simulink model "impedanceExperiments"  (R2019a)
settings: Solver=ode4  StartTime=0.0  StopTime=30  FixedStep=0.01  RelTol=1e-3
libraries: dspswit3 x2
settings Model: Creator=JanAriel  LastModifiedBy=JanAriel
settings SolverCC: AlgebraicLoopSolver=LineSearch

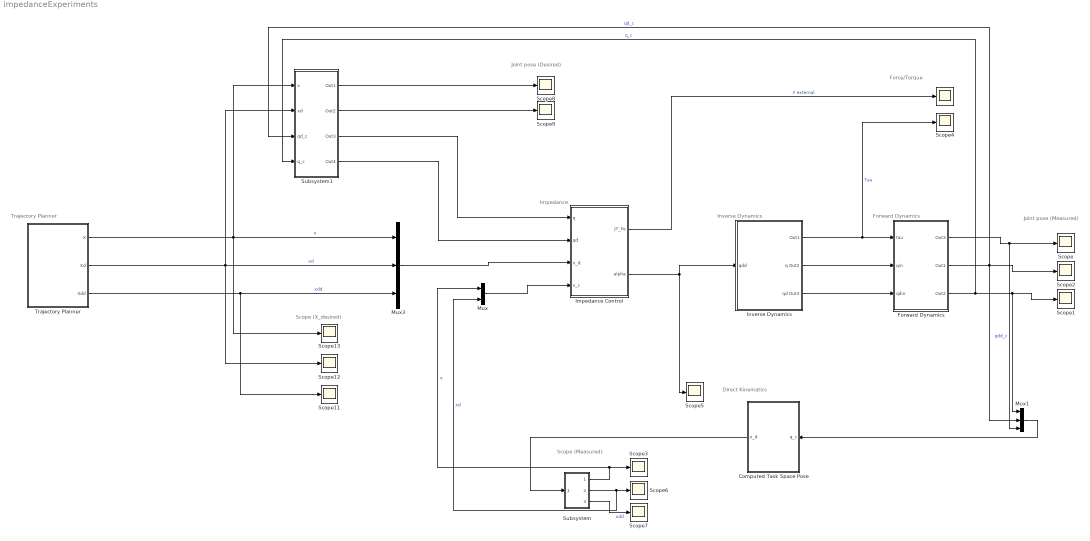
== system impedanceExperiments ==
  note: Joint pose (Desired)
  note: Force/Torque
  note: Joint pose (Measured)
  note: Scope (X_desired)
  note: Scope (Measured)
  note: Trajectory Planner
  note: Forward Dynamics
  note: Inverse Dynamics
  note: Direct Kinematics
  note: Impedance
  " " : Scope
  Computed Task Space Pose : Subsystem
  Forward Dynamics : Subsystem
  Impedance Control : Subsystem
  Inverse Dynamics : Subsystem
  Mux : Mux  Inputs=2
  Mux1 : Mux  Inputs=3
  Mux3 : Mux  Inputs=3
  Scope{,1..9,11..13} (13 alike) : Scope
  Subsystem : Subsystem
  Subsystem1 : Subsystem
  Trajectory Planner : Subsystem
  wires:
  Inverse Dynamics/1(Out1) -> Forward Dynamics/1(tau), Scope4/1  "Tau"
  Inverse Dynamics/2(q Out2) -> Forward Dynamics/2(qin)
  Forward Dynamics/3(Out2) -> Subsystem1/4(q_c), Mux1/1, Scope1/1  "q_c"
  Forward Dynamics/1(Out3) -> Scope/1, Mux1/3  "qdd_c"
  Forward Dynamics/2(Out1) -> Subsystem1/3(qd_c), Mux1/2, Scope2/1  "qd_c"
  Impedance Control/1(JT_Fe) -> " "/1  "F external"
  Trajectory Planner/1(X) -> Subsystem1/1(x), Mux3/1, Scope13/1  "x"
  Trajectory Planner/2(Xd) -> Scope12/1, Mux3/2, Subsystem1/2(xd)  "xd"
  Trajectory Planner/3(Xdd) -> Scope11/1, Mux3/3  "xdd"
  Mux3/1 -> Impedance Control/3(x_d)
  Inverse Dynamics/3(qd Out3) -> Forward Dynamics/3(qdin)
  Computed Task Space Pose/1(x_d) -> Subsystem/1(In1)
  Mux1/1 -> Computed Task Space Pose/1(q_c)
  Impedance Control/2(alpha) -> Scope5/1, Inverse Dynamics/1(qdd)
  Subsystem/1(Out1) -> Scope3/1, Mux/1  "x"
  Subsystem/2(Out2) -> Mux/2, Scope6/1  "xd"
  Subsystem/3(Out3) -> Scope7/1  "xdd"
  Mux/1 -> Impedance Control/4(x_c)
  Subsystem1/1(Out1) -> Scope8/1
  Subsystem1/2(Out2) -> Scope9/1
  Subsystem1/3(Out3) -> Impedance Control/1(q)
  Subsystem1/4(Out4) -> Impedance Control/2(qd)

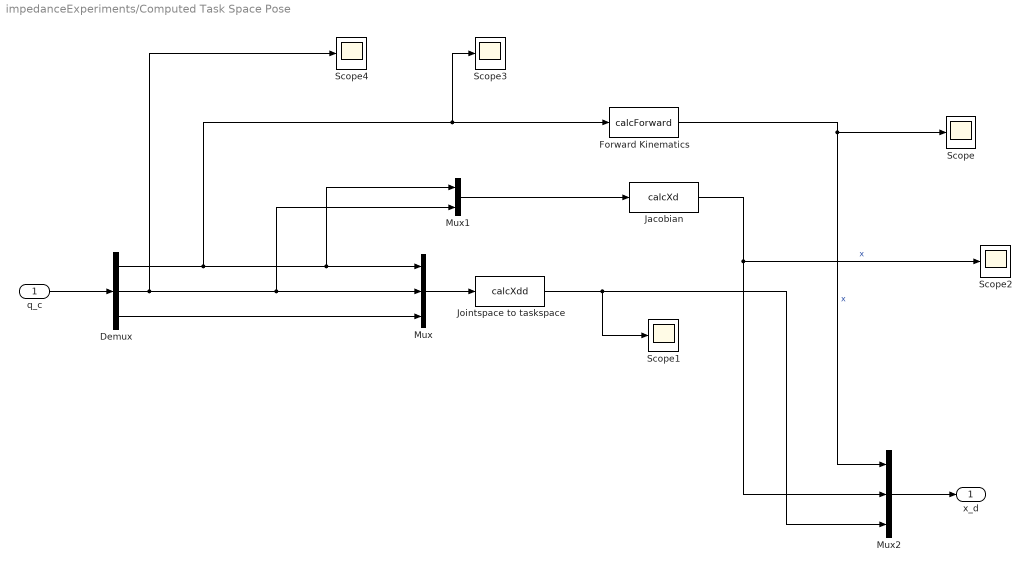
== system impedanceExperiments/Computed Task Space Pose ==
  q_c : Inport
  Demux : Demux  Outputs=3
  Forward Kinematics : MATLABFcn  MATLABFcn=calcForward  Output1D=off
  Jacobian : MATLABFcn  MATLABFcn=calcXd  Output1D=off
  Jointspace to taskspace : MATLABFcn  MATLABFcn=calcXdd  Output1D=off
  Mux : Mux  Inputs=3
  Mux1 : Mux  Inputs=2
  Mux2 : Mux  Inputs=3
  Scope{,1..4} (5 alike) : Scope
  x_d : Outport
  wires:
  q_c/1 -> Demux/1
  Mux/1 -> Jointspace to taskspace/1
  Demux/2 -> Scope4/1, Mux/2, Mux1/2
  Forward Kinematics/1 -> Mux2/1, Scope/1  "x"
  Demux/1 -> Scope3/1, Forward Kinematics/1, Mux/1, Mux1/1
  Mux1/1 -> Jacobian/1
  Demux/3 -> Mux/3
  Jointspace to taskspace/1 -> Scope1/1, Mux2/3
  Mux2/1 -> x_d/1
  Jacobian/1 -> Scope2/1, Mux2/2  "x"

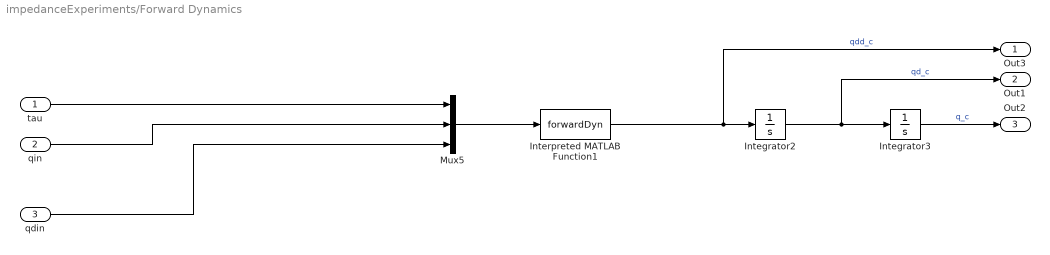
== system impedanceExperiments/Forward Dynamics ==
  tau : Inport
  qin : Inport  Port=2
  qdin : Inport  Port=3
  Integrator2 : Integrator
  Integrator3 : Integrator
  Interpreted MATLAB Function1 : MATLABFcn  MATLABFcn=forwardDyn  Output1D=off
  Mux5 : Mux  Inputs=3
  Out3 : Outport
  Out1 : Outport  Port=2
  Out2 : Outport  Port=3
  wires:
  Integrator2/1 -> Integrator3/1, Out1/1  "qd_c"
  Integrator3/1 -> Out2/1  "q_c"
  Interpreted MATLAB Function1/1 -> Out3/1, Integrator2/1  "qdd_c"
  tau/1 -> Mux5/1
  qin/1 -> Mux5/2
  qdin/1 -> Mux5/3
  Mux5/1 -> Interpreted MATLAB Function1/1

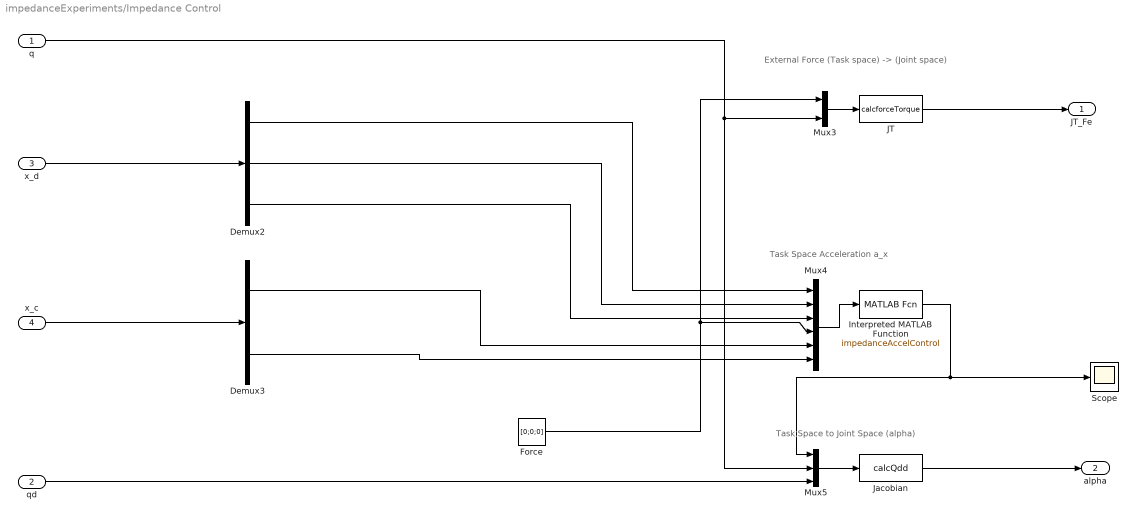
== system impedanceExperiments/Impedance Control ==
  note: Task Space to Joint Space (alpha)
  note: Task Space Acceleration a_x
  note: External Force (Task space) -> (Joint space)
  q : Inport
  qd : Inport  Port=2
  x_d : Inport  Port=3
  x_c : Inport  Port=4
  Demux2 : Demux  Outputs=3
  Demux3 : Demux  Outputs=2
  Force : Constant  Value=[0;0;0]
  Interpreted MATLAB Function : MATLABFcn  MATLABFcn=impedanceAccelControl  Output1D=off
  JT : MATLABFcn  MATLABFcn=calcforceTorque  Output1D=off
  Jacobian : MATLABFcn  MATLABFcn=calcQdd  Output1D=off
  Mux3 : Mux  Inputs=2
  Mux4 : Mux  Inputs=6
  Mux5 : Mux  Inputs=3
  Scope : Scope
  JT_Fe : Outport
  alpha : Outport  Port=2
  wires:
  Demux2/2 -> Mux4/2
  Mux3/1 -> JT/1
  JT/1 -> JT_Fe/1
  Demux2/1 -> Mux4/1
  Demux2/3 -> Mux4/3
  Mux4/1 -> Interpreted MATLAB Function/1
  q/1 -> Mux3/2, Mux5/2
  Mux5/1 -> Jacobian/1
  Interpreted MATLAB Function/1 -> Mux5/1, Scope/1
  Jacobian/1 -> alpha/1
  qd/1 -> Mux5/3
  x_d/1 -> Demux2/1
  Demux3/1 -> Mux4/5
  Demux3/2 -> Mux4/6
  x_c/1 -> Demux3/1
  Force/1 -> Mux3/1, Mux4/4

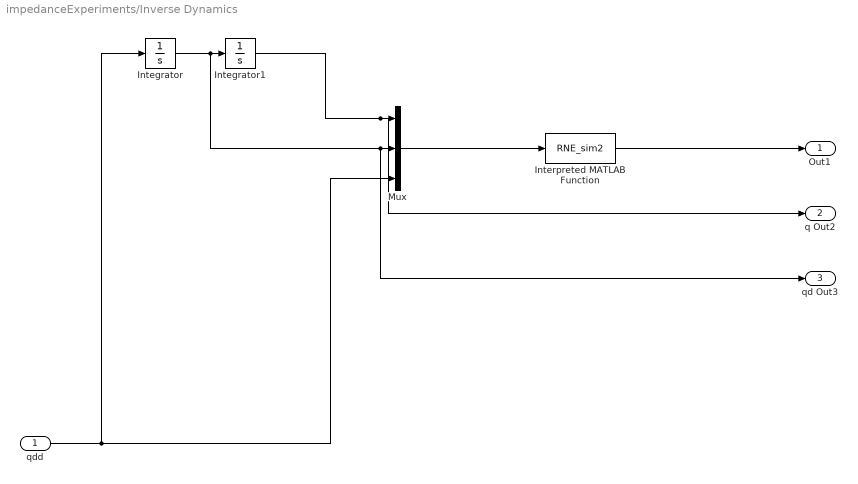
== system impedanceExperiments/Inverse Dynamics ==
  qdd : Inport
  Integrator : Integrator
  Integrator1 : Integrator
  Interpreted MATLAB Function : MATLABFcn  MATLABFcn=RNE_sim2  Output1D=off
  Mux : Mux  Inputs=3
  Out1 : Outport
  q Out2 : Outport  Port=2
  qd Out3 : Outport  Port=3
  wires:
  Mux/1 -> Interpreted MATLAB Function/1
  Interpreted MATLAB Function/1 -> Out1/1
  qdd/1 -> Integrator/1, Mux/3
  Integrator/1 -> qd Out3/1, Mux/2, Integrator1/1
  Integrator1/1 -> q Out2/1, Mux/1

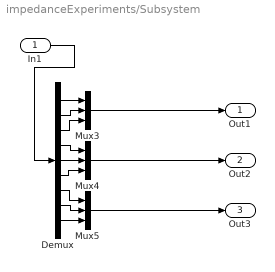
== system impedanceExperiments/Subsystem ==
  In1 : Inport
  Demux : Demux  Outputs=9
  Mux3 : Mux  Inputs=3
  Mux4 : Mux  Inputs=3
  Mux5 : Mux  Inputs=3
  Out1 : Outport
  Out2 : Outport  Port=2
  Out3 : Outport  Port=3
  wires:
  Demux/8 -> Mux5/2
  Demux/7 -> Mux5/1
  Demux/1 -> Mux3/1
  Demux/3 -> Mux3/3
  Demux/9 -> Mux5/3
  Demux/6 -> Mux4/3
  Demux/5 -> Mux4/2
  Demux/4 -> Mux4/1
  Demux/2 -> Mux3/2
  Mux5/1 -> Out3/1
  In1/1 -> Demux/1
  Mux4/1 -> Out2/1
  Mux3/1 -> Out1/1

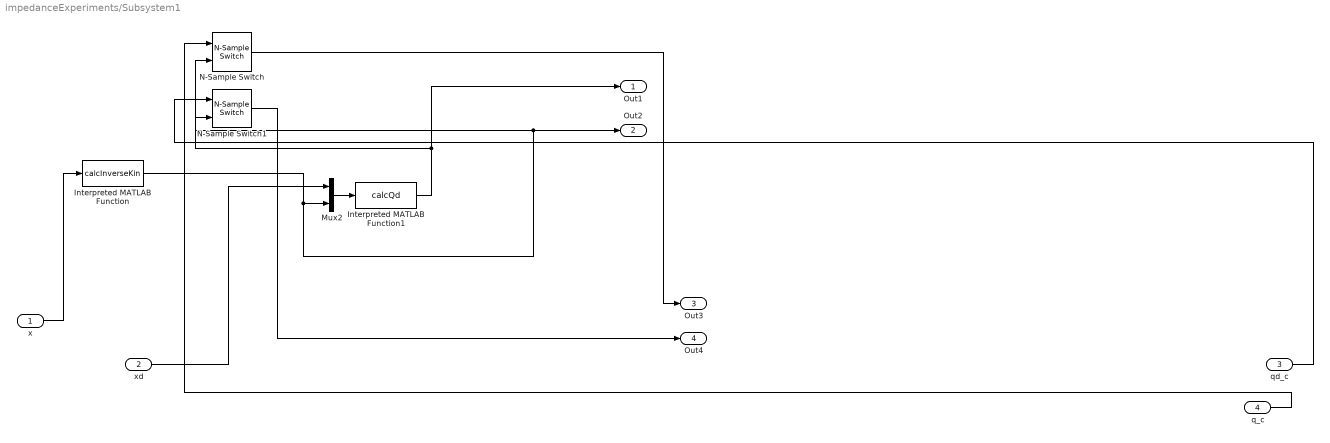
== system impedanceExperiments/Subsystem1 ==
  x : Inport
  xd : Inport  Port=2
  qd_c : Inport  Port=3
  q_c : Inport  Port=4
  Interpreted MATLAB Function : MATLABFcn  MATLABFcn=calcInverseKin  Output1D=off
  Interpreted MATLAB Function1 : MATLABFcn  MATLABFcn=calcQd  Output1D=off
  Mux2 : Mux  Inputs=2
  N-Sample Switch : dspswit3/N-Sample Switch  N=1  reset=off  TriggerType=Rising edge  Ts=0.03
      settings: SourceProductName=DSP System Toolbox  SourceProductBaseCode=DS
  N-Sample Switch1 : dspswit3/N-Sample Switch  N=1  reset=off  TriggerType=Rising edge  Ts=0.03
      settings: SourceProductName=DSP System Toolbox  SourceProductBaseCode=DS
  Out1 : Outport
  Out2 : Outport  Port=2
  Out3 : Outport  Port=3
  Out4 : Outport  Port=4
  wires:
  xd/1 -> Mux2/1
  Interpreted MATLAB Function1/1 -> Out1/1, N-Sample Switch1/2
  N-Sample Switch1/1 -> Out4/1
  Interpreted MATLAB Function/1 -> Out2/1, N-Sample Switch/2, Mux2/2
  Mux2/1 -> Interpreted MATLAB Function1/1
  qd_c/1 -> N-Sample Switch1/1
  N-Sample Switch/1 -> Out3/1
  x/1 -> Interpreted MATLAB Function/1
  q_c/1 -> N-Sample Switch/1

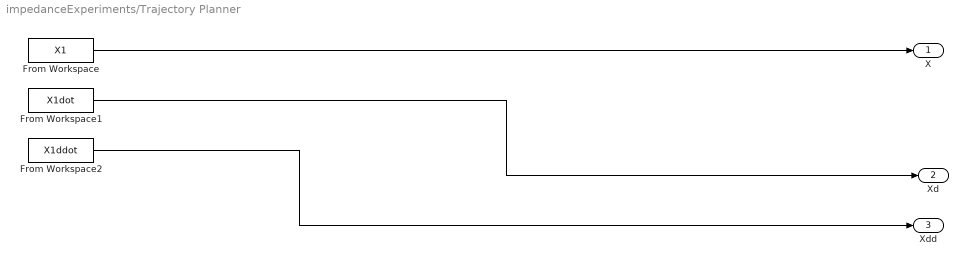
== system impedanceExperiments/Trajectory Planner ==
  From Workspace : FromWorkspace  VariableName=X1  SampleTime=0
  From Workspace1 : FromWorkspace  VariableName=X1dot  SampleTime=0
  From Workspace2 : FromWorkspace  VariableName=X1ddot  SampleTime=0
  X : Outport
  Xd : Outport  Port=2
  Xdd : Outport  Port=3
  wires:
  From Workspace/1 -> X/1
  From Workspace1/1 -> Xd/1
  From Workspace2/1 -> Xdd/1
